simulink model "OffsetNonlinear_a"  (R2019a)
settings: Solver=VariableStepAuto  StartTime=0.0  StopTime=10.0  RelTol=1e-3
values from neighbouring files (symbols this model uses):
  eq = [0, 0, psi_eq, 0]    [offset_dynamics.m]
  K = lqr(A, B, Q, R)    [SimNonlinear.m]    (also in normal_dyn_controller.mat = [-31.6227766017 -46.3910592069 186.459754798 34.6298374135]; offset_dyn_controller.mat = [-31.6227766017 -46.4351184767 187.329434162 34.9118542309]; offset_dynamics.m = lqr(A_sys, B_sys, Q, R))
  motorparams = [kT R r]    [offset_dynamics_params.m]
  params = [l, mp, mc, Ip, Ic, g, f]    [normal_dynamics_params.m]    (also in normal_dynamics_sim.m = normal_dynamics_params(); offset_dynamics.m = offset_dynamics_params(); offset_dynamics_params.m = [l po pu mp md mc Ip Id Ic g f]; offset_dynamics_sim.m = [l po pu mp md mc Ip Id Ic g f])
  x0 = 1    [SimNonlinear.m]    (also in normal_dynamics_sim.m = [0; 0; -pi/4; 0]; offset_dynamics_sim.m = [0; 0; pi; 0])
libraries: simulink x1
settings Model: Creator=Mike Dermksian  LastModifiedBy=Mike Dermksian

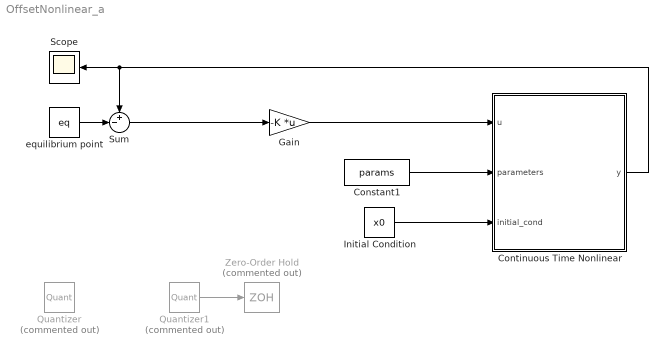
== system OffsetNonlinear_a ==
  Constant1 : Constant  Value=params
  Continuous Time Nonlinear : Subsystem
  Gain : Gain  Gain=-K  Multiplication=Matrix(K*u)
  Initial Condition : Constant  Value=x0
  Quantizer : Quantizer  Commented=on  QuantizationInterval=4/1024
  Quantizer1 : Quantizer  Commented=on  QuantizationInterval=10/256
  Scope : Scope
  Sum : Sum  Inputs=+-|
  Zero-Order Hold : ZeroOrderHold  Commented=on  SampleTime=-1
  equilibrium point : Constant  Value=eq
  wires:
  equilibrium point/1 -> Sum/2
  Continuous Time Nonlinear/1(y) -> Scope/1, Sum/1
  Constant1/1 -> Continuous Time Nonlinear/2(parameters)
  Initial Condition/1 -> Continuous Time Nonlinear/3(initial_cond)
  Sum/1 -> Gain/1
  Quantizer1/1 -> Zero-Order Hold/1
  Gain/1 -> Continuous Time Nonlinear/1(u)

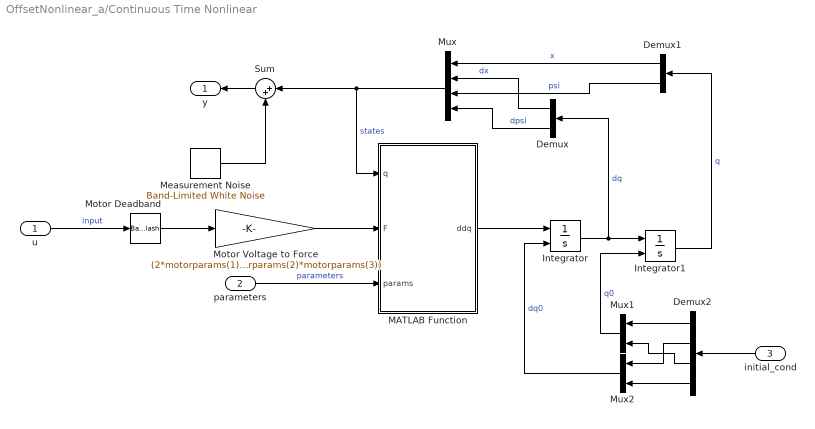
== system OffsetNonlinear_a/Continuous Time Nonlinear ==
  u : Inport
  parameters : Inport  Port=2
  initial_cond : Inport  Port=3
  Demux : Demux  Outputs=2
  Demux1 : Demux  Outputs=2
  Demux2 : Demux
  Integrator : Integrator  InitialConditionSource=external
  Integrator1 : Integrator  InitialConditionSource=external
  MATLAB Function : MATLAB Function  TreatAsAtomicUnit=on
  Measurement Noise : simulink/Sources/Band-Limited White Noise  Cov=[1e-6 1e-6 1e-6 1e-6]  Ts=0.01  seed=[23341]
  Motor Deadband : Backlash
  Motor Voltage to Force : Gain  Gain=(2*motorparams(1))/(motorparams(2)*motorparams(3))
  Mux : Mux
  Mux1 : Mux  Inputs=2
  Mux2 : Mux  Inputs=2
  Sum : Sum  Inputs=|++
  y : Outport
  wires:
  Demux1/1 -> Mux/1  "x"
  Integrator/1 -> Demux/1, Integrator1/1  "dq"
  Integrator1/1 -> Demux1/1  "q"
  Demux2/1 -> Mux1/1
  Mux1/1 -> Integrator1/2  "q0"
  Demux2/4 -> Mux2/2
  Demux1/2 -> Mux/3  "psi"
  Demux/2 -> Mux/4  "dpsi"
  MATLAB Function/1(ddq) -> Integrator/1
  Mux2/1 -> Integrator/2  "dq0"
  Demux2/2 -> Mux2/1
  Demux2/3 -> Mux1/2
  Demux/1 -> Mux/2  "dx"
  u/1 -> Motor Deadband/1  "input"
  initial_cond/1 -> Demux2/1
  Mux/1 -> Sum/1, MATLAB Function/1(q)  "states"
  parameters/1 -> MATLAB Function/3(params)  "parameters"
  Sum/1 -> y/1
  Measurement Noise/1 -> Sum/2
  Motor Voltage to Force/1 -> MATLAB Function/2(F)
  Motor Deadband/1 -> Motor Voltage to Force/1

== matlab function OffsetNonlinear_a/Continuous Time Nonlinear/MATLAB Function ==
  data: q input size=[1 4]; ddq output size=[2 1]; F input; params input size=[1 11]
function ddq = fcn(q, F, params)
ddq = offsetdyn_fun([q(1), q(2), q(3), q(4)], F, params);
